simulink library "robotDynamicsWithContacts_lib_2020"  (R2020b)
settings: Solver=VariableStepAuto  StartTime=0.0  StopTime=10.0  RelTol=1e-3
undefined symbols (not defined in the file or in its folder): contact_config, physics_config, robot_config
libraries: WBToolboxLibrary x9
settings Model: Creator=nunoguedelha  LastModifiedBy=nunoguedelha

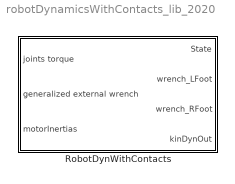
== system robotDynamicsWithContacts_lib_2020 ==
  RobotDynWithContacts : Subsystem  LoadFcn=|  InitFcn=|  mask{robot_config=robot_config, contact_config=contact_config, physics_config=physics_config}
      LoadFcn=|
      | %% initialize the simulation
      | cd(fileparts(which(bdroot)));
      | loadRobotDynamicsWithContactsCB;
      InitFcn=|
      | %% initialize the simulation
      | cd(fileparts(which(bdroot)));
      | initRobotDynamicsWithContactsCB;
      mask DialogControl toggleHighlighting Prompt: Toggle Config Block Highlighting
      mask DialogControl toggleHighlighting Callback:
      | [configBlock, ~] = WBToolbox.BlockInitialization(gcb, gcs);
      | 
      | try
      |     if (strcmp(get_param(configBlock,'HiliteAncestors'),'none'))
      |         hilite_system(configBlock,'find');
      |     else
      |         hilite_system(configBlock,'none');
      |     end
      | catch
      |     error('[%s:ShowConfigBlock:Callback] Failed to process config block name: %s',gcb,configBlock);
      | end
      | 
      | clear configBlock

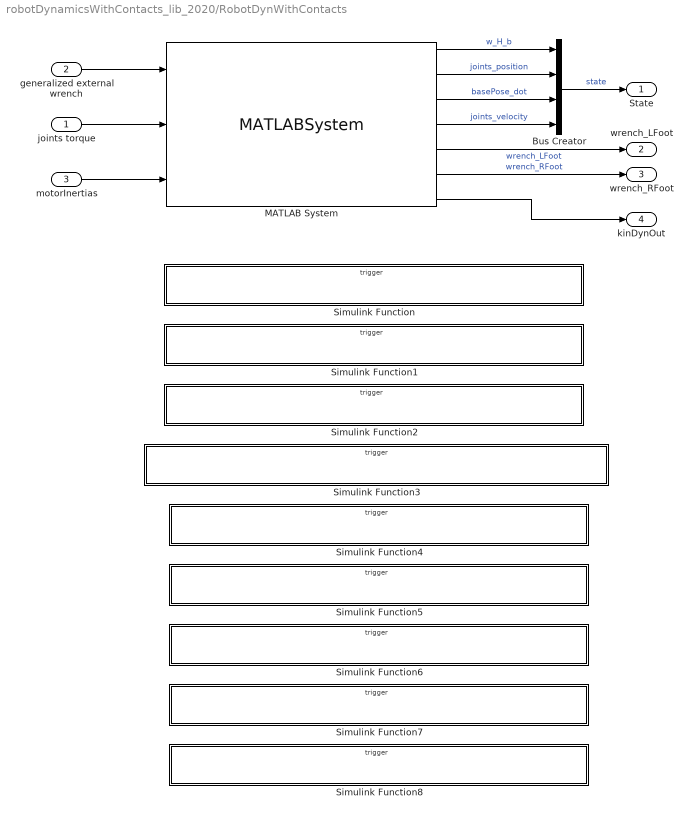
== system robotDynamicsWithContacts_lib_2020/RobotDynWithContacts ==
  joints torque : Inport
  generalized external wrench : Inport  Port=2
  motorInertias : Inport  Port=3
  Bus Creator : BusCreator  Inputs=4
  MATLAB System : MATLABSystem  System=robotDynWC.step_block  robot_config=robot_config  contact_config=contact_config  physics_config=physics_config  OutputBusName=kinDynOut_bus  SimulateUsing=Code generation
      mask Type: robotDynWC.step_block
      mask Display:
      | disp('step_block');
      | port_label('input',1,'generalized_ext_wrench');
      | port_label('input',2,'torque');
      | port_label('input',3,'motorInertias');
      | port_label('output',1,'w_H_b');
      | port_label('output',2,'s');
      | port_label('output',3,'base_pose_dot');
      | port_label('output',4,'s_dot');
      | port_label('output',5,'wrench_left_foot');
      | port_label('output',6,'wrench_right_foot');
      | port_label('output',7,'kinDynOut');
  Simulink Function : Subsystem  TreatAsAtomicUnit=on
  Simulink Function1 : Subsystem  TreatAsAtomicUnit=on
  Simulink Function2 : Subsystem  TreatAsAtomicUnit=on
  Simulink Function3 : Subsystem  TreatAsAtomicUnit=on
  Simulink Function4 : Subsystem  TreatAsAtomicUnit=on
  Simulink Function5 : Subsystem  TreatAsAtomicUnit=on
  Simulink Function6 : Subsystem  TreatAsAtomicUnit=on
  Simulink Function7 : Subsystem  TreatAsAtomicUnit=on
  Simulink Function8 : Subsystem  TreatAsAtomicUnit=on
  State : Outport
  wrench_LFoot : Outport  Port=2
  wrench_RFoot : Outport  Port=3
  kinDynOut : Outport  Port=4
  wires:
  Bus Creator/1 -> State/1  "state"
  MATLAB System/5 -> wrench_LFoot/1  "wrench_LFoot"
  MATLAB System/6 -> wrench_RFoot/1  "wrench_RFoot"
  MATLAB System/1 -> Bus Creator/1  "w_H_b"
  MATLAB System/2 -> Bus Creator/2  "joints_position"
  MATLAB System/3 -> Bus Creator/3  "basePose_dot"
  MATLAB System/4 -> Bus Creator/4  "joints_velocity"
  joints torque/1 -> MATLAB System/2
  generalized external wrench/1 -> MATLAB System/1
  MATLAB System/7 -> kinDynOut/1
  motorInertias/1 -> MATLAB System/3

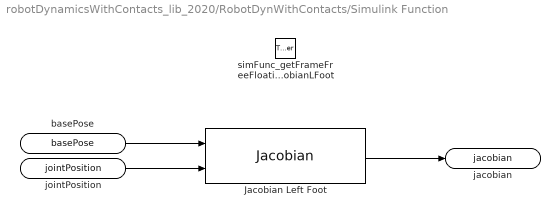
== system robotDynamicsWithContacts_lib_2020/RobotDynWithContacts/Simulink Function ==
  simFunc_getFrameFreeFloatingJacobianLFoot : TriggerPort  TriggerType=function-call  IsSimulinkFunction=on  FunctionName=simFunc_getFrameFreeFloatingJacobianLFoot  FunctionVisibility=scoped  VariantControl=(inherit)
  Jacobian Left Foot : WBToolboxLibrary/Model/Jacobians/Jacobian  frameName=robot_config.robotFrames.LEFT_FOOT
      settings: SourceProductName=WholeBodyToolbox
  basePose : ArgIn  DisableCoverage=on  PortDimensions=[4,4]  ArgumentName=basePose
  jointPosition : ArgIn  Port=2  PortDimensions=[robot_config.N_DOF,1]  ArgumentName=jointPosition
  jacobian : ArgOut  DisableCoverage=on  PortDimensions=[6,6+robot_config.N_DOF]  ArgumentName=jacobian
  wires:
  basePose/1 -> Jacobian Left Foot/1
  jointPosition/1 -> Jacobian Left Foot/2
  Jacobian Left Foot/1 -> jacobian/1

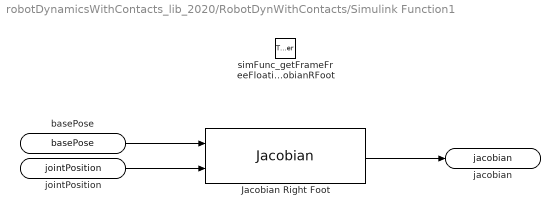
== system robotDynamicsWithContacts_lib_2020/RobotDynWithContacts/Simulink Function1 ==
  simFunc_getFrameFreeFloatingJacobianRFoot : TriggerPort  TriggerType=function-call  IsSimulinkFunction=on  FunctionName=simFunc_getFrameFreeFloatingJacobianRFoot  FunctionVisibility=scoped  VariantControl=(inherit)
  Jacobian Right Foot : WBToolboxLibrary/Model/Jacobians/Jacobian  frameName=robot_config.robotFrames.RIGHT_FOOT
      settings: SourceProductName=WholeBodyToolbox
  basePose : ArgIn  DisableCoverage=on  PortDimensions=[4,4]  ArgumentName=basePose
  jointPosition : ArgIn  Port=2  PortDimensions=[robot_config.N_DOF,1]  ArgumentName=jointPosition
  jacobian : ArgOut  DisableCoverage=on  PortDimensions=[6,6+robot_config.N_DOF]  ArgumentName=jacobian
  wires:
  basePose/1 -> Jacobian Right Foot/1
  jointPosition/1 -> Jacobian Right Foot/2
  Jacobian Right Foot/1 -> jacobian/1

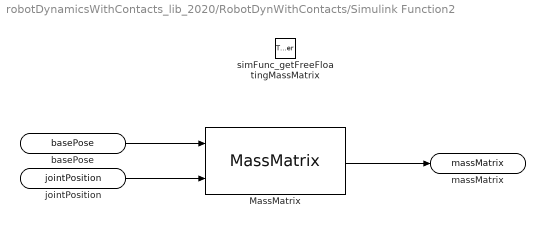
== system robotDynamicsWithContacts_lib_2020/RobotDynWithContacts/Simulink Function2 ==
  simFunc_getFreeFloatingMassMatrix : TriggerPort  TriggerType=function-call  IsSimulinkFunction=on  FunctionName=simFunc_getFreeFloatingMassMatrix  FunctionVisibility=scoped  VariantControl=(inherit)
  MassMatrix : WBToolboxLibrary/Model/Dynamics/MassMatrix
      settings: SourceProductName=WholeBodyToolbox
  basePose : ArgIn  DisableCoverage=on  PortDimensions=[4,4]  ArgumentName=basePose
  jointPosition : ArgIn  Port=2  PortDimensions=[robot_config.N_DOF,1]  ArgumentName=jointPosition
  massMatrix : ArgOut  DisableCoverage=on  PortDimensions=[6+robot_config.N_DOF,6+robot_config.N_DOF]  ArgumentName=massMatrix
  wires:
  basePose/1 -> MassMatrix/1
  jointPosition/1 -> MassMatrix/2
  MassMatrix/1 -> massMatrix/1

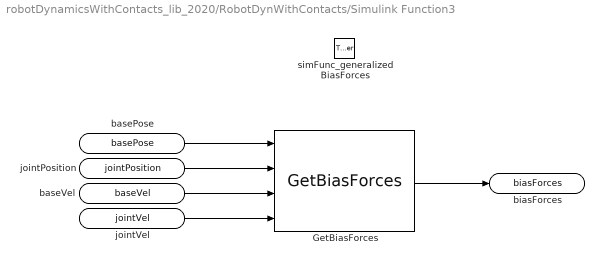
== system robotDynamicsWithContacts_lib_2020/RobotDynWithContacts/Simulink Function3 ==
  simFunc_generalizedBiasForces : TriggerPort  TriggerType=function-call  IsSimulinkFunction=on  FunctionName=simFunc_generalizedBiasForces  FunctionVisibility=scoped  VariantControl=(inherit)
  GetBiasForces : WBToolboxLibrary/Model/Dynamics/GetBiasForces
      settings: SourceProductName=WholeBodyToolbox
  basePose : ArgIn  DisableCoverage=on  PortDimensions=[4,4]  ArgumentName=basePose
  jointPosition : ArgIn  Port=2  PortDimensions=[robot_config.N_DOF,1]  ArgumentName=jointPosition
  baseVel : ArgIn  Port=3  PortDimensions=[6,1]  ArgumentName=baseVel
  jointVel : ArgIn  Port=4  PortDimensions=[robot_config.N_DOF,1]  ArgumentName=jointVel
  biasForces : ArgOut  DisableCoverage=on  PortDimensions=[6+robot_config.N_DOF,1]  ArgumentName=biasForces
  wires:
  basePose/1 -> GetBiasForces/1
  jointPosition/1 -> GetBiasForces/2
  GetBiasForces/1 -> biasForces/1
  baseVel/1 -> GetBiasForces/3
  jointVel/1 -> GetBiasForces/4

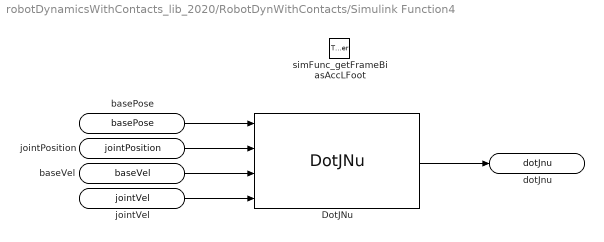
== system robotDynamicsWithContacts_lib_2020/RobotDynWithContacts/Simulink Function4 ==
  simFunc_getFrameBiasAccLFoot : TriggerPort  TriggerType=function-call  IsSimulinkFunction=on  FunctionName=simFunc_getFrameBiasAccLFoot  FunctionVisibility=scoped  VariantControl=(inherit)
  DotJNu : WBToolboxLibrary/Model/Jacobians/DotJNu  frameName=robot_config.robotFrames.LEFT_FOOT
      settings: SourceProductName=WholeBodyToolbox
  basePose : ArgIn  DisableCoverage=on  PortDimensions=[4,4]  ArgumentName=basePose
  jointPosition : ArgIn  Port=2  PortDimensions=[robot_config.N_DOF,1]  ArgumentName=jointPosition
  baseVel : ArgIn  Port=3  PortDimensions=[6,1]  ArgumentName=baseVel
  jointVel : ArgIn  Port=4  PortDimensions=[robot_config.N_DOF,1]  ArgumentName=jointVel
  dotJnu : ArgOut  DisableCoverage=on  PortDimensions=[6,1]  ArgumentName=dotJnu
  wires:
  DotJNu/1 -> dotJnu/1
  jointPosition/1 -> DotJNu/2
  basePose/1 -> DotJNu/1
  baseVel/1 -> DotJNu/3
  jointVel/1 -> DotJNu/4

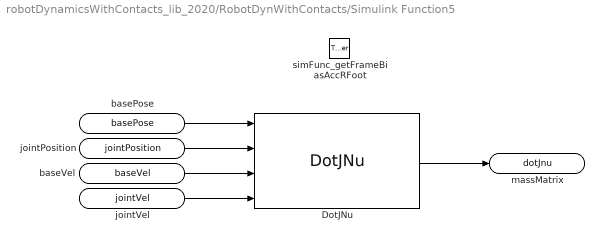
== system robotDynamicsWithContacts_lib_2020/RobotDynWithContacts/Simulink Function5 ==
  simFunc_getFrameBiasAccRFoot : TriggerPort  TriggerType=function-call  IsSimulinkFunction=on  FunctionName=simFunc_getFrameBiasAccRFoot  FunctionVisibility=scoped  VariantControl=(inherit)
  DotJNu : WBToolboxLibrary/Model/Jacobians/DotJNu  frameName=robot_config.robotFrames.RIGHT_FOOT
      settings: SourceProductName=WholeBodyToolbox
  basePose : ArgIn  DisableCoverage=on  PortDimensions=[4,4]  ArgumentName=basePose
  jointPosition : ArgIn  Port=2  PortDimensions=[robot_config.N_DOF,1]  ArgumentName=jointPosition
  baseVel : ArgIn  Port=3  PortDimensions=[6,1]  ArgumentName=baseVel
  jointVel : ArgIn  Port=4  PortDimensions=[robot_config.N_DOF,1]  ArgumentName=jointVel
  massMatrix : ArgOut  DisableCoverage=on  PortDimensions=[6,1]  ArgumentName=dotJnu
  wires:
  DotJNu/1 -> massMatrix/1
  jointPosition/1 -> DotJNu/2
  basePose/1 -> DotJNu/1
  baseVel/1 -> DotJNu/3
  jointVel/1 -> DotJNu/4

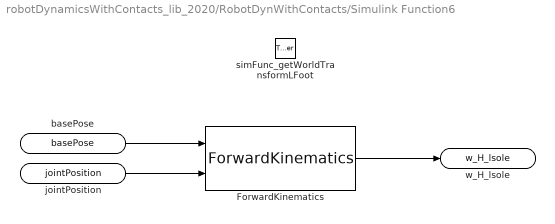
== system robotDynamicsWithContacts_lib_2020/RobotDynWithContacts/Simulink Function6 ==
  simFunc_getWorldTransformLFoot : TriggerPort  TriggerType=function-call  IsSimulinkFunction=on  FunctionName=simFunc_getWorldTransformLFoot  FunctionVisibility=scoped  VariantControl=(inherit)
  ForwardKinematics : WBToolboxLibrary/Model/Kinematics/ForwardKinematics  frameName=robot_config.robotFrames.LEFT_FOOT
      settings: SourceProductName=WholeBodyToolbox
  basePose : ArgIn  DisableCoverage=on  PortDimensions=[4,4]  ArgumentName=basePose
  jointPosition : ArgIn  Port=2  PortDimensions=[robot_config.N_DOF,1]  ArgumentName=jointPosition
  w_H_lsole : ArgOut  DisableCoverage=on  PortDimensions=[4,4]  ArgumentName=w_H_lsole
  wires:
  basePose/1 -> ForwardKinematics/1
  jointPosition/1 -> ForwardKinematics/2
  ForwardKinematics/1 -> w_H_lsole/1

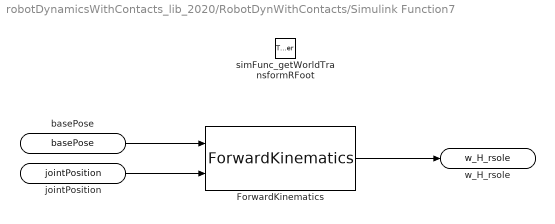
== system robotDynamicsWithContacts_lib_2020/RobotDynWithContacts/Simulink Function7 ==
  simFunc_getWorldTransformRFoot : TriggerPort  TriggerType=function-call  IsSimulinkFunction=on  FunctionName=simFunc_getWorldTransformRFoot  FunctionVisibility=scoped  VariantControl=(inherit)
  ForwardKinematics : WBToolboxLibrary/Model/Kinematics/ForwardKinematics  frameName=robot_config.robotFrames.RIGHT_FOOT
      settings: SourceProductName=WholeBodyToolbox
  basePose : ArgIn  DisableCoverage=on  PortDimensions=[4,4]  ArgumentName=basePose
  jointPosition : ArgIn  Port=2  PortDimensions=[robot_config.N_DOF,1]  ArgumentName=jointPosition
  w_H_rsole : ArgOut  DisableCoverage=on  PortDimensions=[4,4]  ArgumentName=w_H_rsole
  wires:
  basePose/1 -> ForwardKinematics/1
  jointPosition/1 -> ForwardKinematics/2
  ForwardKinematics/1 -> w_H_rsole/1

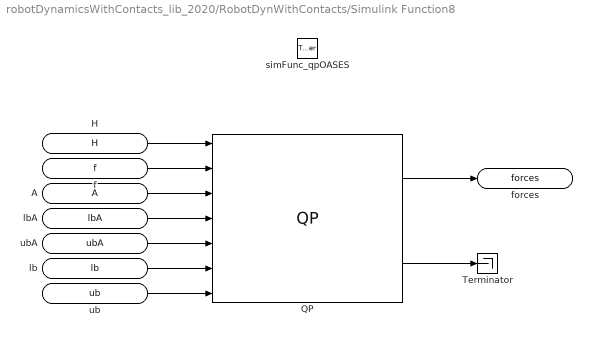
== system robotDynamicsWithContacts_lib_2020/RobotDynWithContacts/Simulink Function8 ==
  simFunc_qpOASES : TriggerPort  TriggerType=function-call  IsSimulinkFunction=on  FunctionName=simFunc_qpOASES  FunctionVisibility=scoped  VariantControl=(inherit)
  QP : WBToolboxLibrary/Utilities/QP  lbA=on  ubA=on  lb=on  ub=on  computeObjVal=off  stopIfFails=off
      settings: SourceProductName=WholeBodyToolbox
  Terminator : Terminator
  H : ArgIn  DisableCoverage=on  PortDimensions=[3*contact_config.total_num_vertices,3*contact_config.total_num_vertices]  ArgumentName=H
  f : ArgIn  Port=2  PortDimensions=[3*contact_config.total_num_vertices,1]  ArgumentName=f
  A : ArgIn  Port=3  PortDimensions=[5*contact_config.total_num_vertices,3*contact_config.total_num_vertices]  ArgumentName=A
  lbA : ArgIn  Port=4  PortDimensions=[5*contact_config.total_num_vertices,1]  ArgumentName=lbA
  ubA : ArgIn  Port=5  PortDimensions=[5*contact_config.total_num_vertices,1]  ArgumentName=ubA
  lb : ArgIn  Port=6  PortDimensions=[3*contact_config.total_num_vertices,1]  ArgumentName=lb
  ub : ArgIn  Port=7  PortDimensions=[3*contact_config.total_num_vertices,1]  ArgumentName=ub
  forces : ArgOut  DisableCoverage=on  PortDimensions=[3*contact_config.total_num_vertices,1]  ArgumentName=forces
  wires:
  H/1 -> QP/1
  f/1 -> QP/2
  QP/1 -> forces/1
  A/1 -> QP/3
  lbA/1 -> QP/4
  QP/2 -> Terminator/1
  ubA/1 -> QP/5
  lb/1 -> QP/6
  ub/1 -> QP/7
